simulink model "GonzalezGC21210380P3LA"  (R2024b)
settings: Solver=ode15s  StartTime=0.0  StopTime=10  MaxStep=1E-3  RelTol=1e-3
settings DataIOCC: ReturnWorkspaceOutputs=off  TimeSaveName=t
settings DebuggingCC: AlgebraicLoopMsg=none  ArtificialAlgebraicLoopMsg=none  BlockPriorityViolationMsg=error  MinStepSizeMsg=error  MaxConsecutiveZCsMsg=none  OperatingPointInterfaceChecksumMismatchMsg=none

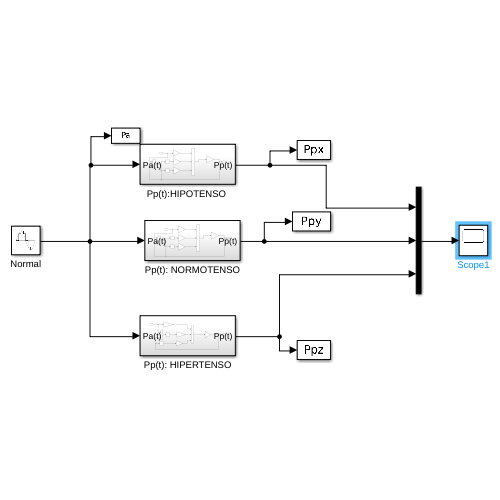
[thumbnail: Simulink's stored preview of the top-level diagram]
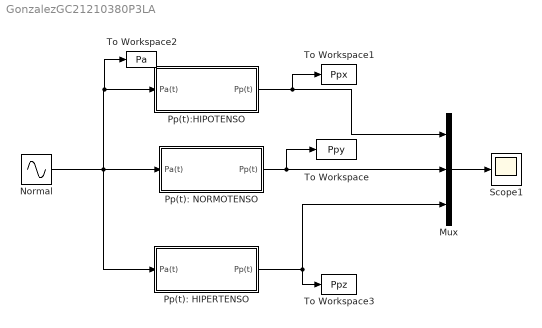
== system GonzalezGC21210380P3LA ==
  Mux : Mux  Inputs=3
  Normal : Sin  Bias=0.8  Frequency=(2*pi)*(95/60)  SampleTime=0.001
  Pp(t): HIPERTENSO : Subsystem
  Pp(t): NORMOTENSO : Subsystem
  "Pp(t):HIPOTENSO " : Subsystem
  Scope1 : Scope
  To Workspace : ToWorkspace  VariableName=Ppy  SampleTime=-1
  To Workspace1 : ToWorkspace  VariableName=Ppx  SampleTime=-1
  To Workspace2 : ToWorkspace  VariableName=Pa  SaveFormat=Timeseries  SampleTime=-1
  To Workspace3 : ToWorkspace  VariableName=Ppz  SampleTime=-1
  wires:
  Normal/1 -> Pp(t): NORMOTENSO/1(Pa(t)), Pp(t): HIPERTENSO/1(Pa(t)), To Workspace2/1, "Pp(t):HIPOTENSO "/1(Pa(t))
  "Pp(t):HIPOTENSO "/1(Pp(t)) -> To Workspace1/1, Mux/1
  Pp(t): HIPERTENSO/1(Pp(t)) -> Mux/3, To Workspace3/1
  Pp(t): NORMOTENSO/1(Pp(t)) -> To Workspace/1, Mux/2
  Mux/1 -> Scope1/1

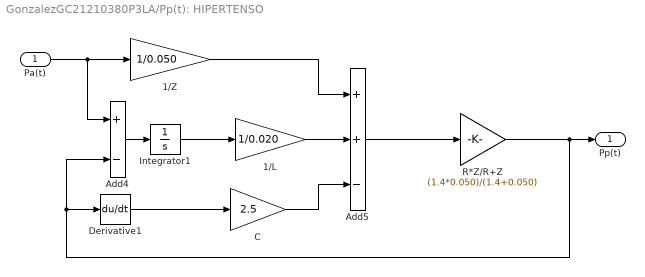
== system GonzalezGC21210380P3LA/Pp(t): HIPERTENSO ==
  Pa(t) : Inport
  1/L : Gain  Gain=1/0.020
  1/Z : Gain  Gain=1/0.050
  Add4 : Sum  Inputs=+-
  Add5 : Sum  Inputs=++-
  C : Gain  Gain=2.5
  Derivative1 : Derivative
  Integrator1 : Integrator
  R*Z/R+Z : Gain  Gain=(1.4*0.050)/(1.4+0.050)
  Pp(t) : Outport
  wires:
  R*Z/R+Z/1 -> Derivative1/1, Add4/2, Pp(t)/1
  Pa(t)/1 -> Add4/1, 1/Z/1
  Derivative1/1 -> C/1
  1/L/1 -> Add5/2
  C/1 -> Add5/3
  Integrator1/1 -> 1/L/1
  Add4/1 -> Integrator1/1
  Add5/1 -> R*Z/R+Z/1
  1/Z/1 -> Add5/1

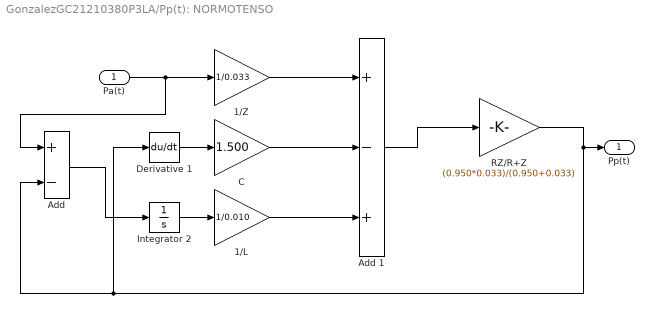
== system GonzalezGC21210380P3LA/Pp(t): NORMOTENSO ==
  Pa(t) : Inport
  1/L : Gain  Gain=1/0.010
  1/Z : Gain  Gain=1/0.033
  Add : Sum  Inputs=+-
  Add 1 : Sum  Inputs=+-+
  C : Gain  Gain=1.500
  Derivative 1 : Derivative
  Integrator 2 : Integrator
  RZ/R+Z : Gain  Gain=(0.950*0.033)/(0.950+0.033)
  Pp(t) : Outport
  wires:
  Add 1/1 -> RZ/R+Z/1
  C/1 -> Add 1/2
  RZ/R+Z/1 -> Derivative 1/1, Add/2, Pp(t)/1
  Pa(t)/1 -> Add/1, 1/Z/1
  Add/1 -> Integrator 2/1
  Integrator 2/1 -> 1/L/1
  1/L/1 -> Add 1/3
  Derivative 1/1 -> C/1
  1/Z/1 -> Add 1/1

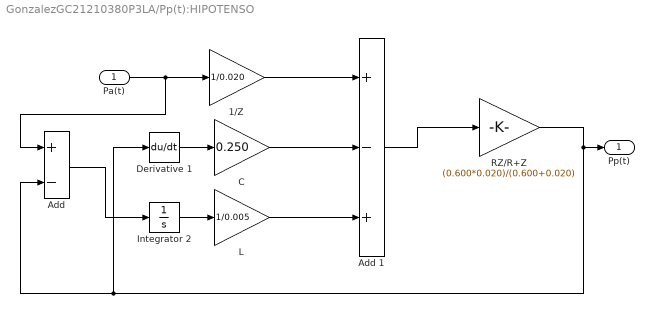
== system GonzalezGC21210380P3LA/Pp(t):HIPOTENSO  ==
  Pa(t) : Inport
  1/Z : Gain  Gain=1/0.020
  Add : Sum  Inputs=+-
  Add 1 : Sum  Inputs=+-+
  C : Gain  Gain=0.250
  Derivative 1 : Derivative
  Integrator 2 : Integrator
  L : Gain  Gain=1/0.005
  RZ/R+Z : Gain  Gain=(0.600*0.020)/(0.600+0.020)
  Pp(t) : Outport
  wires:
  Add 1/1 -> RZ/R+Z/1
  Pa(t)/1 -> Add/1, 1/Z/1
  1/Z/1 -> Add 1/1
  C/1 -> Add 1/2
  L/1 -> Add 1/3
  Derivative 1/1 -> C/1
  Integrator 2/1 -> L/1
  RZ/R+Z/1 -> Derivative 1/1, Add/2, Pp(t)/1
  Add/1 -> Integrator 2/1
